simulink model "general_Test"  (R2022b)
settings: Solver=VariableStepAuto  StartTime=0.0  StopTime=10.0  RelTol=1e-3
settings Model: Creator=umber  LastModifiedBy=umber
settings DataIOCC: ExternalInput=a.getElement('current')  LoadExternalInput=on
settings ModelReferenceCC: EnableRefExpFcnMdlSchedulingChecks=on

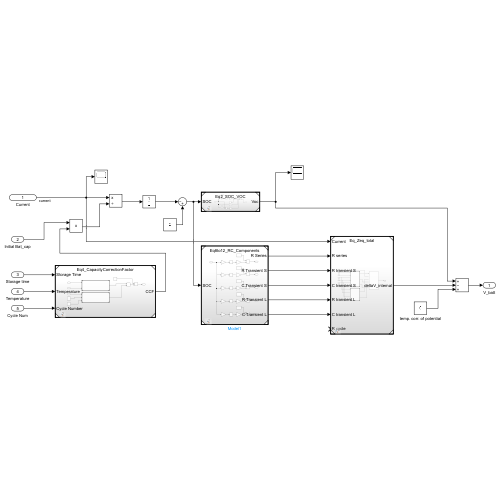
[thumbnail: Simulink's stored preview of the top-level diagram]
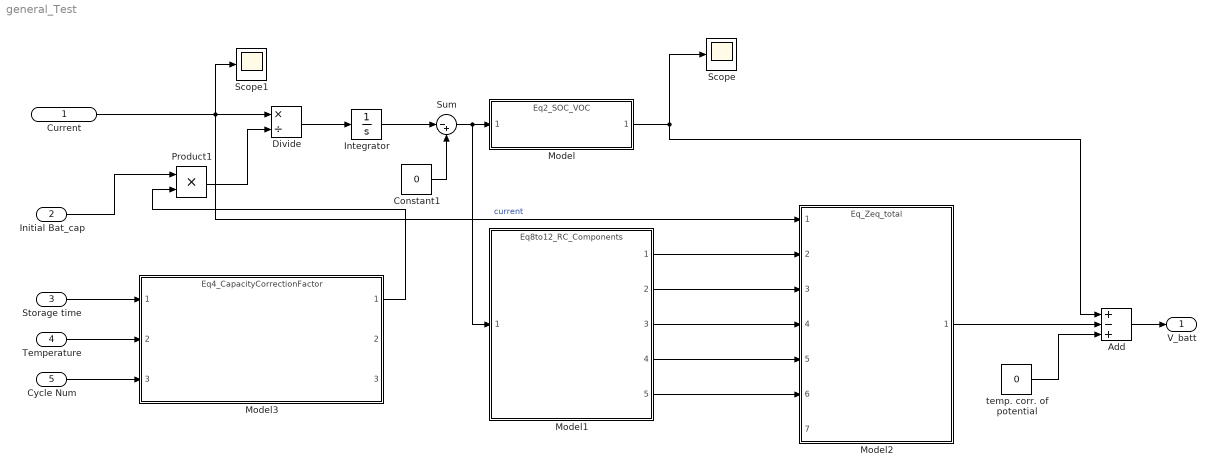
== system general_Test ==
  Current : Inport
  Initial Bat_cap : Inport  Port=2
  Storage time : Inport  Port=3
  Temperature : Inport  Port=4
  Cycle Num : Inport  Port=5
  Add : Sum  Inputs=+-+
  Constant1 : Constant  Value=0
  Divide : Product  Inputs=*/
  Integrator : Integrator
  Model : ModelReference  ModelNameDialog=Eq2_SOC_VOC.slx  SimulationMode=Normal  ModelReferenceVersion=1.3
  Model1 : ModelReference  ModelNameDialog=Eq8to12_RC_Components  SimulationMode=Normal  ModelReferenceVersion=1.1
  Model2 : ModelReference  ModelNameDialog=Eq_Zeq_total.slx  SimulationMode=Normal  ModelReferenceVersion=1.3
  Model3 : ModelReference  ModelNameDialog=Eq4_CapacityCorrectionFactor.slx  SimulationMode=Normal  ModelReferenceVersion=2.0
  Product1 : Product
  Scope : Scope
  Scope1 : Scope
  Sum : Sum  Inputs=|-+
  temp. corr. of potential : Constant  Value=0
  V_batt : Outport
  wires:
  Divide/1 -> Integrator/1
  Integrator/1 -> Sum/1
  Sum/1 -> Model1/1, Model/1
  Current/1 -> Scope1/1, Model2/1, Divide/1  "current"
  Constant1/1 -> Sum/2
  Model/1 -> Add/1, Scope/1
  Model1/1 -> Model2/2
  Model1/2 -> Model2/3
  Model1/3 -> Model2/4
  Model1/4 -> Model2/5
  Model1/5 -> Model2/6
  Model2/1 -> Add/2
  Add/1 -> V_batt/1
  temp. corr. of potential/1 -> Add/3
  Model3/1 -> Product1/2
  Product1/1 -> Divide/2
  Initial Bat_cap/1 -> Product1/1
  Cycle Num/1 -> Model3/3
  Temperature/1 -> Model3/2
  Storage time/1 -> Model3/1
